simulink model "main"  (R2024a)
settings: Solver=FixedStepAuto  StartTime=0.0  StopTime=T  FixedStep=dt  RelTol=1e-3
values from neighbouring files (symbols this model uses):
  ctrl_dt = 1/1e3    (= 0.001)    [main_slx.m]
  W_init = zeros(x_num)    [main_slx.m]
  x = [0;0;0;0]    [main_slx.m]
  X_init = 1    [main_slx.m]
settings Model: Creator=dding  LastModifiedBy=DDing
settings RTWCC: GPUComputeCapability=3.5

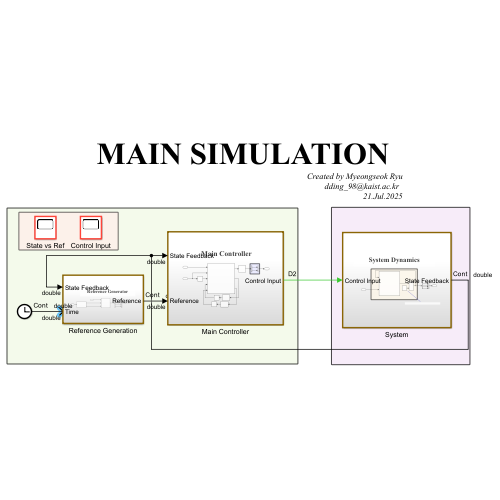
[thumbnail: Simulink's stored preview of the top-level diagram]
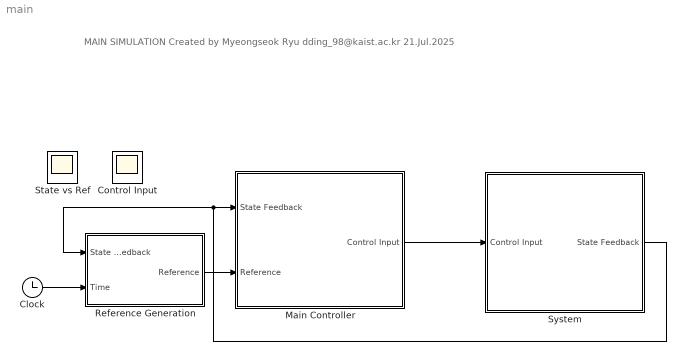
== system main ==
  note: MAIN SIMULATION
      | Created by Myeongseok Ryu
      | dding_98@kaist.ac.kr
      | 21.Jul.2025
  Clock : Clock
  Control Input : Scope
      settings: Floating=on
  Main Controller : Subsystem
  Reference Generation : Subsystem
  State vs Ref : Scope
      settings: Floating=on
  System : Subsystem
  wires:
  Clock/1 -> Reference Generation/2(Time)
  Reference Generation/1(Reference) -> Main Controller/2(Reference)
  Main Controller/1(Control Input) -> System/1(Control Input)
  System/1(State Feedback) -> Main Controller/1(State Feedback), Reference Generation/1(State Feedback)

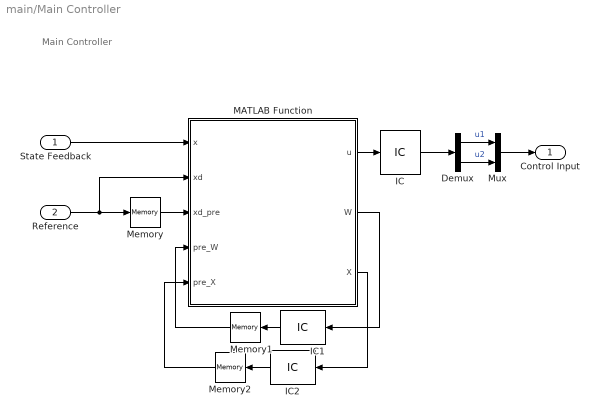
== system main/Main Controller ==
  note: Main Controller
  State Feedback : Inport
  Reference : Inport  Port=2
  Demux : Demux  Outputs=2
  IC : InitialCondition  Value=u
  IC1 : InitialCondition  Value=W_init
  IC2 : InitialCondition  Value=X_init
  MATLAB Function : MATLAB Function  TreatAsAtomicUnit=on  SystemSampleTime=ctrl_dt
  Memory : Memory
  Memory1 : Memory
  Memory2 : Memory
  Mux : Mux  Inputs=2
  Control Input : Outport
  wires:
  Reference/1 -> MATLAB Function/2(xd), Memory/1
  MATLAB Function/1(u) -> IC/1
  State Feedback/1 -> MATLAB Function/1(x)
  Mux/1 -> Control Input/1
  Demux/1 -> Mux/1  "u1"
  Demux/2 -> Mux/2  "u2"
  IC/1 -> Demux/1
  Memory/1 -> MATLAB Function/3(xd_pre)
  MATLAB Function/2(W) -> IC1/1
  Memory1/1 -> MATLAB Function/4(pre_W)
  IC1/1 -> Memory1/1
  MATLAB Function/3(X) -> IC2/1
  IC2/1 -> Memory2/1
  Memory2/1 -> MATLAB Function/5(pre_X)

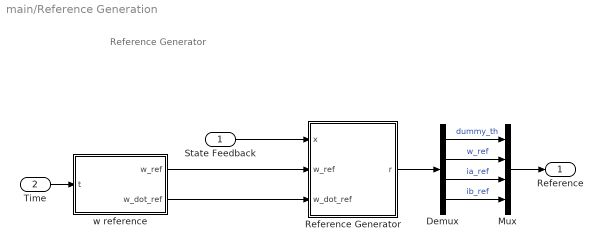
== system main/Reference Generation ==
  note: Reference Generator
  State Feedback : Inport
  Time : Inport  Port=2
  Demux : Demux
  Mux : Mux
  Reference Generator : MATLAB Function  TreatAsAtomicUnit=on
  w reference : MATLAB Function  TreatAsAtomicUnit=on
  Reference : Outport
  wires:
  State Feedback/1 -> Reference Generator/1(x)
  Reference Generator/1(r) -> Demux/1
  Mux/1 -> Reference/1
  Demux/1 -> Mux/1  "dummy_th"
  Demux/2 -> Mux/2  "w_ref"
  Demux/3 -> Mux/3  "ia_ref"
  Time/1 -> w reference/1(t)
  w reference/1(w_ref) -> Reference Generator/2(w_ref)
  w reference/2(w_dot_ref) -> Reference Generator/3(w_dot_ref)
  Demux/4 -> Mux/4  "ib_ref"

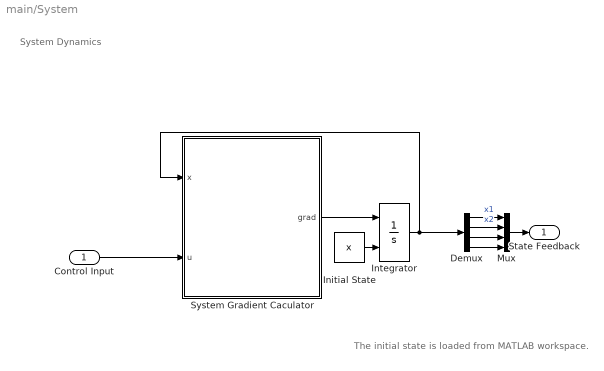
== system main/System ==
  note: The initial state is loaded from MATLAB workspace.
  note: System Dynamics
  Control Input : Inport
  Demux : Demux
  Initial State : Constant  Value=x
  Integrator : Integrator  InitialConditionSource=external
  Mux : Mux
  System Gradient Caculator : MATLAB Function  TreatAsAtomicUnit=on
  State Feedback : Outport
  wires:
  System Gradient Caculator/1(grad) -> Integrator/1
  Integrator/1 -> System Gradient Caculator/1(x), Demux/1
  Initial State/1 -> Integrator/2
  Mux/1 -> State Feedback/1
  Control Input/1 -> System Gradient Caculator/2(u)
  Demux/1 -> Mux/1  "x1"
  Demux/2 -> Mux/2  "x2"
  Demux/3 -> Mux/3
  Demux/4 -> Mux/4

== matlab function main/System/System Gradient Caculator ==
  data: x input; u input; grad output
function grad = fcn(x, u)
    th = x(1);  % theta
    w = x(2);  % theta dot
    ia = x(3);  % Ia
    ib = x(4);  % Ib

    trq_d = 0;
    
    %%
    % L = .66e-3;    % Inductance (mH)
    L = .66;
    R = 0.251;     % Resistance (Ohm)
    J = 3.24e-5;   % Inertia (kg.m^2)
    Phi = 16.8e-3; % Flux (Wb)
    P = 4;         % Pole pairs
    fv = 2e-3;     % Viscous friction (N.m.s/rad)
    
    %% 
    trq = -(3/2)*P*Phi*sin(P*th)*ia + (3/2)*P*Phi*cos(P*th)*ib;

    %%
    grad = [
        w;
        (1/J)*(trq - fv*w + trq_d);
        (1/L)*(u(1) - R*ia + P*Phi*w*sin(P*th));
        (1/L)*(u(2) - R*ib - P*Phi*w*cos(P*th))
    ];
end

== matlab function main/Reference Generation/Reference Generator ==
  data: x input; w_ref input; r output; w_dot_ref input
function r = fcn(x, w_ref, w_dot_ref)
    th = x(1);  % theta
    w = x(2);  % theta dot
    ia = x(3);  % Ia
    ib = x(4);  % Ib

    %%
    % L = .66e-3;    % Inductance (mH)
    L = .66;
    R = 0.251;     % Resistance (Ohm)
    J = 3.24e-5;   % Inertia (kg.m^2)
    Phi = 16.8e-3; % Flux (Wb)
    P = 4;         % Pole pairs
    fv = 2e-3;     % Viscous friction (N.m.s/rad)
    est_tau_L = 0; % we do not estimate disturbance!
    
    %%
    tau_ref = J * w_dot_ref + fv * w_ref + est_tau_L;
    ia_ref = -(2/3)*tau_ref*sin(P*th)/P/Phi;
    ib_ref = +(2/3)*tau_ref*cos(P*th)/P/Phi;
    
    % Appetizer
    r = [
        0;
        w_ref;
        ia_ref;
        ib_ref;
    ];

== matlab function main/Reference Generation/w reference ==
  data: t input; w_ref output; w_dot_ref output
function [w_ref, w_dot_ref]  = fcn(t)

    %%
    start_t = 1;
    duration = 1;
    end_value = 300;

    %%
    if t<start_t
        w_ref = 0;
        w_dot_ref = 0;
    elseif t<start_t+duration
        w_ref = end_value/duration * (t-start_t);
        w_dot_ref = end_value/duration;
    else
        w_ref = end_value;
        w_dot_ref = 0;
    end

end

== matlab function main/Main Controller/MATLAB Function ==
  data: x input; u output; xd input; xd_pre input; ctrl_dt parameter; W output; pre_W input; pre_X input; X output
function [u, W, X] = fcn(x, xd, xd_pre, ctrl_dt, pre_W, pre_X)
    %%
    % x = [th, w, ia, ib]
    
%%
    dt = ctrl_dt;
    R = diag([1, 1])*1e-3;
    inv_R = inv(R);  % input weight matrix

    %%
    L = .66;
    R = 0.251;     % Resistance (Ohm)
    J = 3.24e-5;   % Inertia (kg.m^2)
    Phi = 16.8e-3; % Flux (Wb)
    P = 4;         % Pole pairs
    fv = 2e-3;     % Viscous friction (N.m.s/rad)

    xd_dot = (xd - xd_pre) / dt;
    ud = [
        L*xd_dot(3)+R*xd(3) - P*Phi*xd(2)*sin(P*x(1));
        L*xd_dot(4)+R*xd(4) - P*Phi*xd(2)*cos(P*x(1));
    ];

    %% 
    L = .66;
    B = [
        0, 0;
        1/L, 0; 
        0, 1/L
        ];

    SDC = SDCmotor(x, xd);  % System Dynamics Coefficient

    %%
    W = zeros(3);
    X = 0;
    coder.extrinsic('NCM_init')
    [W,X,optDone] = LMI_solve(pre_W, pre_X, SDC, B, inv_R, dt)
    
    %%
    e = x - xd;
    u = ud - inv_R * B' * inv(W) * e(2:end);  % control input

end


function SDC = SDCmotor(x,xd)

    %%
    % L = .66e-3;    % Inductance (mH)
    L = .66;
    R = 0.251;     % Resistance (Ohm)
    J = 3.24e-5;   % Inertia (kg.m^2)
    Phi = 16.8e-3; % Flux (Wb)
    P = 4;         % Pole pairs
    fv = 2e-3;     % Viscous friction (N.m.s/rad)

    %%
    a21 = 1/J * (-(3/2)*P*Phi) * ...
        (-intXcosY(x(3),xd(3), x(1),xd(1), P) + ...
        intXsinY(x(4),xd(4), x(1),xd(1), P));
    a23 = 1/J * (-(3/2)*P*Phi) * ...
        intXsinY(1,1, x(1),xd(1), P);
    a24 = 1/J * (+(3/2)*P*Phi) * ...
        intXcosY(1,1, x(1),xd(1), P);

    a31 = 1/L*P^2*Phi * ...
        intXcosY(x(2),xd(2), x(1),xd(1), P);
    a41 = 1/L*P^2*Phi * ...
        intXsinY(x(2),xd(2), x(1),xd(1), P);

    a32 = 1/L*P*Phi * ...
        intXsinY(1,1, x(1),xd(1), P);
    a42 = 1/L*P*Phi * ...
        intXcosY(1,1, x(1),xd(1), P);

    %%
    SDC = [
        -fv/J a23 a24;
        a32 -R/L 0;
        a42 0 -R/L
    ];

    for i = 1:1:3
        for j = 1:1:3
            if isnan(SDC(i,j))
                SDC(i,j) = 0;
            end
        end
    end
end

function z = intXsinY(x1,x2, y1,y2, a)
    z = 1/(a*(y1-y2)) * (-cos(a*y1)*x1 + cos(a*y2)*x2) + (x1-x2)/(a*(y1-y2))^2 * (sin(a*y1) - sin(a*y2));
end

function z = intXcosY(x1,x2, y1,y2, a)
    z = 1/(a*(y1-y2)) * (sin(a*y1)*x1 - sin(a*y2)*x2) + (x1-x2)/(a*(y1-y2))^2 * (-cos(a*y1) + cos(a*y2));
end
